simulink model "Lorenca"  (R2021b)
settings: Solver=FixedStepAuto  StartTime=0.0  StopTime=25  FixedStep=0.001  RelTol=1e-3
settings Model: Creator=Tymon  LastModifiedBy=Tymon

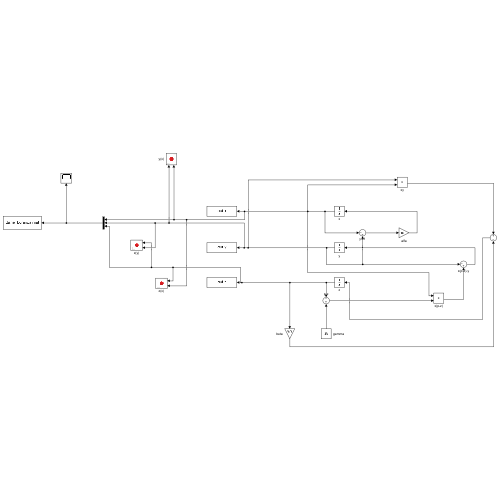
[thumbnail: Simulink's stored preview of the top-level diagram]
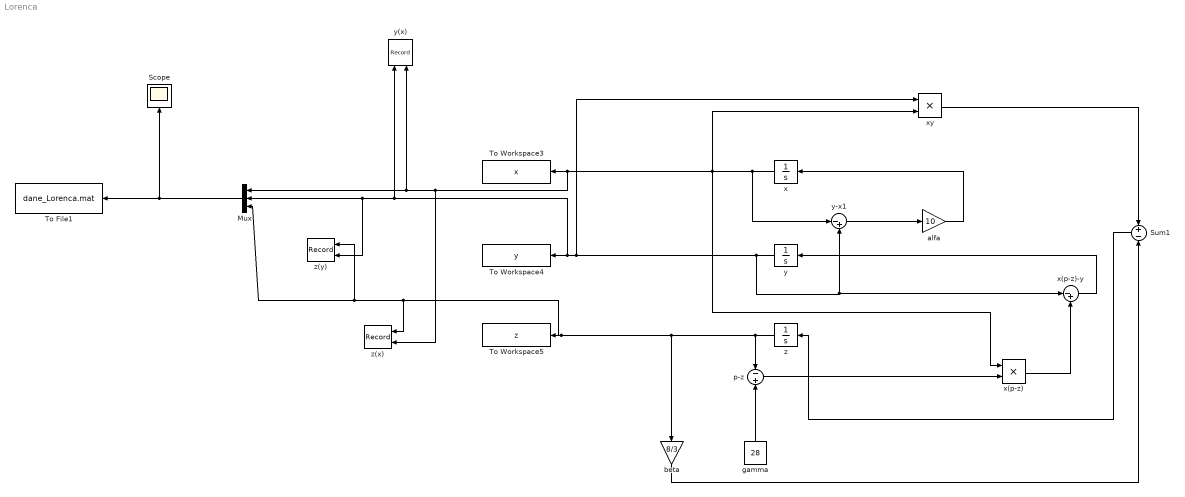
== system Lorenca ==
  Mux : Mux  Inputs=3
  Scope : Scope
  Sum1 : Sum  Inputs=+-
  To File1 : ToFile  Filename=dane_Lorenca.mat  SaveFormat=Timeseries
  To Workspace3 : ToWorkspace  VariableName=x  SampleTime=-1
  To Workspace4 : ToWorkspace  VariableName=y  SampleTime=-1
  To Workspace5 : ToWorkspace  VariableName=z  SampleTime=-1
  alfa : Gain  Gain=10
  beta : Gain  Gain=8/3
  gamma : Constant  Value=28
  p-z : Sum  Inputs=-+
  x : Integrator  InitialCondition=1
  x(p-z) : Product
  x(p-z)-y : Sum  Inputs=|-+
  xy : Product
  y : Integrator  InitialCondition=1
  y(x) : Record  FileSettingsInternal="{\"entries\":[{\"content\":{\"excelSettings\":{\"content\":{},\"type\":\"Streamout.ExcelSettings\"}},\"type\":\"Streamout.FileSettingStorage\",\"uuid\":\"64fce77f-5805-450d-95d6-90c1208abcc3\"}],\"packageUris\":[\"http://schema.mathworks.com/mf0/streamout_blocks/R2020a\"],\"version\":\"1.0\"}"  Layout=[1 1]  SignalsInternal="{\"entries\":[{\"content\":{\"signals\":[{\"content\":{\"blockPath\":[\"Lorenca/y(x)\"],\"channel\":[],\"dimensions\":[1],\"domain\":\"Lorenca/y(x)\",\"lineColor\":\"#a2142f\",\"plots\":[],\"port\":1,\"sid\":[\"\"],\"signalID\":36,\"signalName\":\"y\"},\"type\":\"RecordBlkView.Signal\",\"uuid\":\"c8b8e10f-ff32-4cc5-bae7-40749901c2af\"},{\"content\":{\"blockPath\":[\"Lorenca/y(x)\"],\"channel\":[],\"dimensions\":[1],\"domain\":\"Lorenca/y(x)\",\"lineColor\":\"#139fff\",\"plots\":[],\"port\":2,\"sid\":[\"\"],\"signalID\":40,\"signalName\":\"x\"},\"type\":\"RecordBlkView.Signal\",\"uuid\":\"a958353f-577d-4a73-812f-e6df10b992ab\"}]},\"type\":\"RecordBlkView.InputSignals\",\"uuid\":\"60857ce1-1af0-4b60-b6a6-a2fb32291185\"}],\"packageUris\":[\"http://schema.mathworks.com/mf0/streamout_blocks/R2020a\"],\"version\":\"1.0\"}"  VisualizationBindings="{\"xyplotplugin\":{\"info\":[{\"series\":[],\"subplotID\":1}]}}"  CompatibilityTag=XY
  y-x1 : Sum  Inputs=|-+
  z : Integrator  InitialCondition=1
  z(x) : Record  FileSettingsInternal="{\"entries\":[{\"content\":{\"excelSettings\":{\"content\":{},\"type\":\"Streamout.ExcelSettings\"}},\"type\":\"Streamout.FileSettingStorage\",\"uuid\":\"54b0b319-51f5-4966-93f1-6551f585f869\"}],\"packageUris\":[\"http://schema.mathworks.com/mf0/streamout_blocks/R2020a\"],\"version\":\"1.0\"}"  Layout=[1 1]  SignalsInternal="{\"entries\":[{\"content\":{\"signals\":[{\"content\":{\"blockPath\":[\"Lorenca/z(x)\"],\"channel\":[],\"dimensions\":[1],\"domain\":\"Lorenca/z(x)\",\"lineColor\":\"#ff6929\",\"plots\":[],\"port\":1,\"sid\":[\"\"],\"signalID\":44,\"signalName\":\"z\"},\"type\":\"RecordBlkView.Signal\",\"uuid\":\"a311e66f-41ea-457f-af34-27304f722236\"},{\"content\":{\"blockPath\":[\"Lorenca/z(x)\"],\"channel\":[],\"dimensions\":[1],\"domain\":\"Lorenca/z(x)\",\"lineColor\":\"#b746ff\",\"plots\":[],\"port\":2,\"sid\":[\"\"],\"signalID\":48,\"signalName\":\"x\"},\"type\":\"RecordBlkView.Signal\",\"uuid\":\"9bd5bf98-7168-49dc-8f3e-f8cea359633e\"}]},\"type\":\"RecordBlkView.InputSignals\",\"uuid\":\"4dcdb7e4-1604-46c4-9959-01bc02b072ba\"}],\"packageUris\":[\"http://schema.mathworks.com/mf0/streamout_blocks/R2020a\"],\"version\":\"1.0\"}"  VisualizationBindings="{\"xyplotplugin\":{\"info\":[{\"series\":[],\"subplotID\":1}]}}"  CompatibilityTag=XY
  z(y) : Record  FileSettingsInternal="{\"entries\":[{\"content\":{\"excelSettings\":{\"content\":{},\"type\":\"Streamout.ExcelSettings\"}},\"type\":\"Streamout.FileSettingStorage\",\"uuid\":\"a038a1cc-6167-4cc2-a98b-f89a6f46003e\"}],\"packageUris\":[\"http://schema.mathworks.com/mf0/streamout_blocks/R2020a\"],\"version\":\"1.0\"}"  Layout=[1 1]  SignalsInternal="{\"entries\":[{\"content\":{\"signals\":[{\"content\":{\"blockPath\":[\"Lorenca/z(y)\"],\"channel\":[],\"dimensions\":[1],\"domain\":\"Lorenca/z(y)\",\"lineColor\":\"#64d413\",\"plots\":[],\"port\":1,\"sid\":[\"\"],\"signalID\":52,\"signalName\":\"z\"},\"type\":\"RecordBlkView.Signal\",\"uuid\":\"84d232ba-0032-4bc5-b509-1bec6fadcfd9\"},{\"content\":{\"blockPath\":[\"Lorenca/z(y)\"],\"channel\":[],\"dimensions\":[1],\"domain\":\"Lorenca/z(y)\",\"lineColor\":\"#ff13a6\",\"plots\":[],\"port\":2,\"sid\":[\"\"],\"signalID\":56,\"signalName\":\"y\"},\"type\":\"RecordBlkView.Signal\",\"uuid\":\"10a8f8b9-53cc-4e10-bb06-d84df555447b\"}]},\"type\":\"RecordBlkView.InputSignals\",\"uuid\":\"15f753bc-48a7-456a-9b18-fb93bcbabd0b\"}],\"packageUris\":[\"http://schema.mathworks.com/mf0/streamout_blocks/R2020a\"],\"version\":\"1.0\"}"  VisualizationBindings="{\"xyplotplugin\":{\"info\":[{\"series\":[],\"subplotID\":1}]}}"  CompatibilityTag=XY
  wires:
  x/1 -> y-x1/1, xy/2, x(p-z)/1, z(x)/2, y(x)/2, Mux/1, To Workspace3/1
  y/1 -> xy/1, y(x)/1, z(y)/2, Mux/2, To Workspace4/1, y-x1/2, x(p-z)-y/1
  z/1 -> beta/1, z(x)/1, z(y)/1, Mux/3, To Workspace5/1, p-z/1
  y-x1/1 -> alfa/1
  alfa/1 -> x/1
  gamma/1 -> p-z/2
  p-z/1 -> x(p-z)/2
  x(p-z)/1 -> x(p-z)-y/2
  x(p-z)-y/1 -> y/1
  beta/1 -> Sum1/2
  xy/1 -> Sum1/1
  Sum1/1 -> z/1
  Mux/1 -> To File1/1, Scope/1
